simulink model "breakingDownIntoComponents"  (R2025a)
settings: Solver=VariableStepAuto  StartTime=0.0  StopTime=10.0  RelTol=1e-3
undefined symbols (not defined in the file): V
libraries: SignalEditorBlockLib x1
settings Model: Creator=JPIRES3  LastModifiedBy=JPIRES3

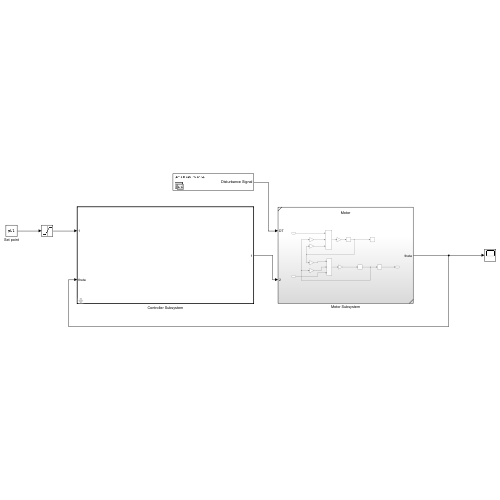
[thumbnail: Simulink's stored preview of the top-level diagram]
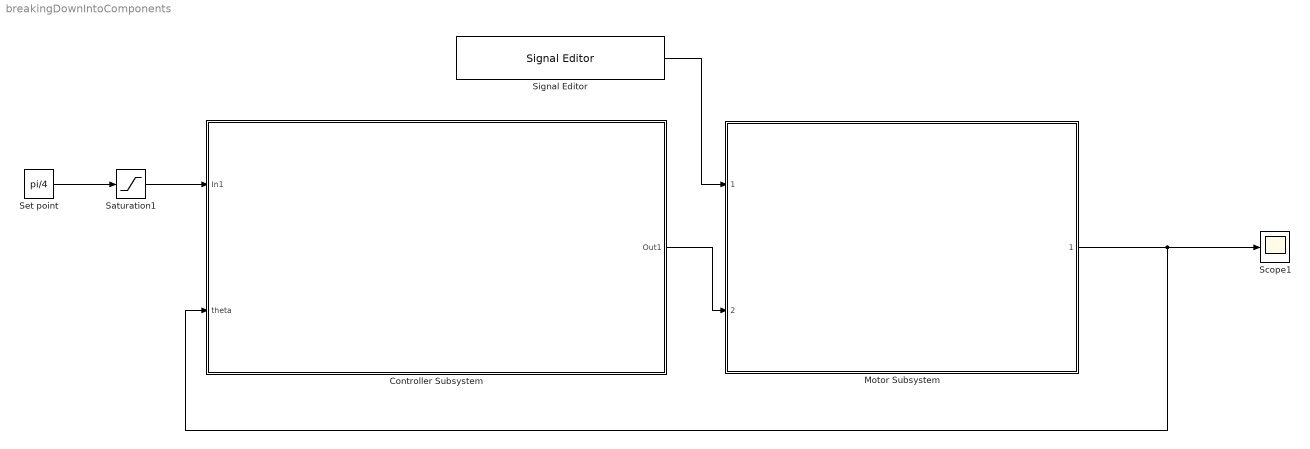
== system breakingDownIntoComponents ==
  Controller Subsystem : Subsystem  TreatAsAtomicUnit=on  mask{kp=9.39, ki=7.33, Ts=0.01}
      mask prompts: kp "proportional Gain"; ki "Integral Gain"; Ts "Sample Time"
  Motor Subsystem : Subsystem  ReferencedSubsystem=Motor
  Saturation1 : Saturate  UpperLimit=pi/4  LowerLimit=-pi/4
  Scope1 : Scope
      settings: ActiveDisplayYMinimum=-0.11554258584712604  ActiveDisplayYMaximum=1.0398832726241345
  Set point : Constant  Value=pi/4
  Signal Editor : SignalEditorBlockLib/Signal Editor  FileName=C:\Users\jpires3\Documents\Matlab-projects\Module 3 - Introduction to subsystems\Disturbance.mat  ActiveScenario=SmallDisturbance  ActiveSignal=Disturbance Signal  IsBus=off  OutputBusObjectStr=Bus: BusObject  SampleTime=0  ZeroCross=off  OutputAfterFinalValue=Setting to zero  Unit=inherit  PreserveSignalName=on  ApplySigPropsToAllScenarios=on  ApplySigPropsToAllSignals=off  SignalPropertySource=Dialog parameters
  wires:
  Set point/1 -> Saturation1/1
  Signal Editor/1 -> Motor Subsystem/1
  Controller Subsystem/1(Out1) -> Motor Subsystem/2
  Saturation1/1 -> Controller Subsystem/1(In1)
  Motor Subsystem/1 -> Controller Subsystem/2(theta), Scope1/1

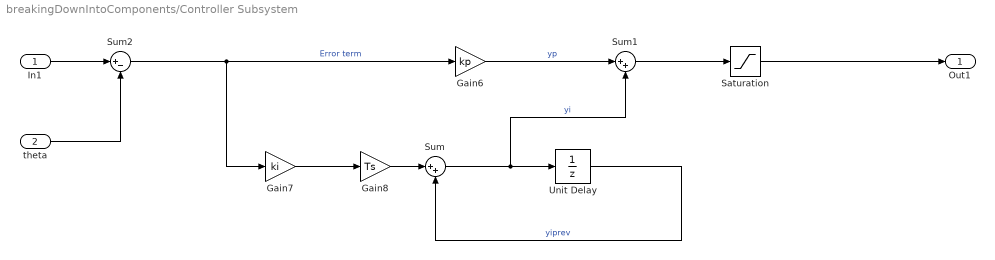
== system breakingDownIntoComponents/Controller Subsystem ==
  In1 : Inport
  theta : Inport  Port=2
  Gain6 : Gain  Gain=kp
  Gain7 : Gain  Gain=ki
  Gain8 : Gain  Gain=Ts
  Saturation : Saturate  UpperLimit=V  LowerLimit=-V
  Sum : Sum  Inputs=|++
  Sum1 : Sum  Inputs=|++
  Sum2 : Sum  Inputs=|+-
  Unit Delay : UnitDelay  InitialCondition=1  SampleTime=Ts  HasFrameUpgradeWarning=on
  Out1 : Outport
  wires:
  Gain8/1 -> Sum/1
  Sum/1 -> Sum1/2, Unit Delay/1  "yi"
  Sum1/1 -> Saturation/1
  Unit Delay/1 -> Sum/2  "yiprev"
  In1/1 -> Sum2/1
  Gain6/1 -> Sum1/1  "yp"
  Sum2/1 -> Gain7/1, Gain6/1  "Error term"
  Saturation/1 -> Out1/1
  Gain7/1 -> Gain8/1
  theta/1 -> Sum2/2
